simulink model "planar_kinctrl1"  (R2020b)
settings: Solver=VariableStepAuto  StartTime=0.0  StopTime=10  RelTol=1e-3
values from neighbouring files (symbols this model uses):
  q0 = [pi -pi/2 -pi/2]    [planar_mdl.m]
libraries: roblocks x3
settings Model: Creator=lucas  LastModifiedBy=lucas

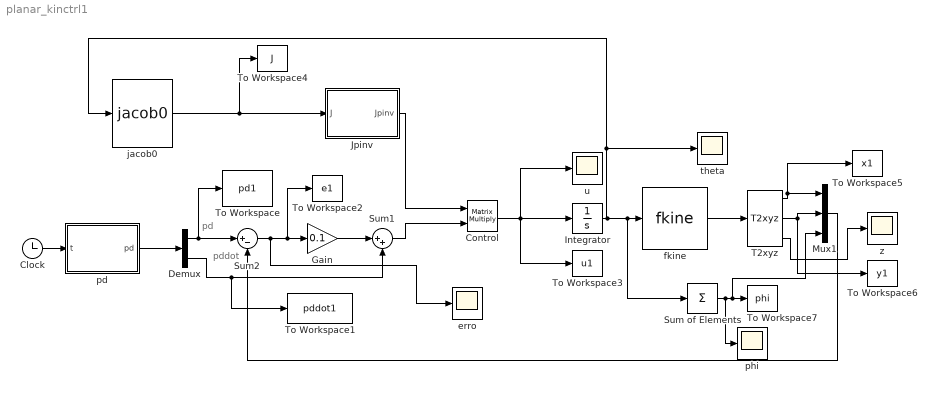
== system planar_kinctrl1 ==
  note: pd
  note: pddot
  Clock : Clock
  Control : Product  Inputs=**  Multiplication=Matrix(*)
  Demux : Demux  Outputs=2
  Gain : Gain  Gain=0.1
  Integrator : Integrator  InitialCondition=q0
  Jpinv : MATLAB Function  TreatAsAtomicUnit=on
  Mux1 : Mux  Inputs=3
  Sum of Elements : Sum  Inputs=+
  Sum1 : Sum  Inputs=|++
  Sum2 : Sum  Inputs=|+-
  T2xyz : roblocks/Toolbox/T2xyz
  To Workspace : ToWorkspace  VariableName=pd1  SaveFormat=Timeseries  SampleTime=-1
  To Workspace1 : ToWorkspace  VariableName=pddot1  SaveFormat=Timeseries  SampleTime=-1
  To Workspace2 : ToWorkspace  VariableName=e1  SaveFormat=Timeseries  SampleTime=-1
  To Workspace3 : ToWorkspace  VariableName=u1  SaveFormat=Timeseries  SampleTime=-1
  To Workspace4 : ToWorkspace  VariableName=J  SaveFormat=Timeseries  SampleTime=-1
  To Workspace5 : ToWorkspace  VariableName=x1  SaveFormat=Timeseries  SampleTime=-1
  To Workspace6 : ToWorkspace  VariableName=y1  SaveFormat=Timeseries  SampleTime=-1
  To Workspace7 : ToWorkspace  VariableName=phi  SaveFormat=Timeseries  SampleTime=-1
  erro : Scope
  fkine : roblocks/Arm/fkine  robot=planar
  "jacob0 " : roblocks/Arm/jacob0   robot=planar
  pd : MATLAB Function  TreatAsAtomicUnit=on
  phi : Scope
  theta : Scope
  u : Scope
  z : Scope
  wires:
  Clock/1 -> pd/1(t)
  Demux/2 -> To Workspace1/1, Sum1/2
  pd/1(pd) -> Demux/1
  Demux/1 -> Sum2/1, To Workspace/1
  Sum2/1 -> erro/1, To Workspace2/1, Gain/1
  Gain/1 -> Sum1/1
  Sum1/1 -> Control/2
  "jacob0 "/1 -> Jpinv/1(J), To Workspace4/1
  fkine/1 -> T2xyz/1
  T2xyz/2 -> Mux1/2, To Workspace6/1
  T2xyz/1 -> Mux1/1, To Workspace5/1
  Mux1/1 -> Sum2/2
  Integrator/1 -> Sum of Elements/1, fkine/1, "jacob0 "/1, theta/1
  Control/1 -> u/1, Integrator/1, To Workspace3/1
  T2xyz/3 -> z/1
  Sum of Elements/1 -> phi/1, Mux1/3, To Workspace7/1
  Jpinv/1(Jpinv) -> Control/1

== matlab function planar_kinctrl1/Jpinv ==
  data: J input; Jpinv output
function Jpinv = Jpinv(J)
    J1 = J(1:2,1:3);
    J2 = J(6,1:3);
    J = [J1;J2];
    Jpinv = pinv(J);

== matlab function planar_kinctrl1/pd ==
  data: t input; pd output
function pd  = fcn(t)

xd = [0.25*(1-cos(pi*t)) 0.25*(2+sin(pi*t)) sin(pi*t/24)]';
xddot = [0.25*pi*sin(pi*t) 0.25*pi*cos(pi*t) (pi/24)*cos(pi*t/24)]';

pd=[xd;xddot];
